simulink model "Prod_mod"  (R2016b)
settings: Solver=VariableStepAuto  StartTime=0.0  StopTime=9000  MaxStep=0.01  RelTol=1e-4  EnableMultiTasking=on
undefined symbols (not defined in the file or in its folder): DiscIntNeverNeededParam
libraries: simulink x2
settings Model: Creator=Joseph Lee  LastModifiedBy=Joseph Lee
settings DataIOCC: LimitDataPoints=on  SaveOutput=off  SaveTime=off
settings OptimizationCC: ExpressionDepthLimit=2147483647  LifeSpan=1
settings DebuggingCC: UnderspecifiedInitializationDetection=Classic  MergeDetectMultiDrivingBlocksExec=none  FcnCallInpInsideContextMsg=warning  AllowSymbolicDim=off  StateNameClashWarn=warning  SFUnexpectedBacktrackingDiag=warning  SFNoUnconditionalDefaultTransitionDiag=warning  SFExecutionAtInitializationDiag=none
settings GRTTargetCC: TargetLangStandard=C89/C90 (ANSI)  GeneratePreprocessorConditionals=Disable all  CombineOutputUpdateFcns=off  GRTInterface=on

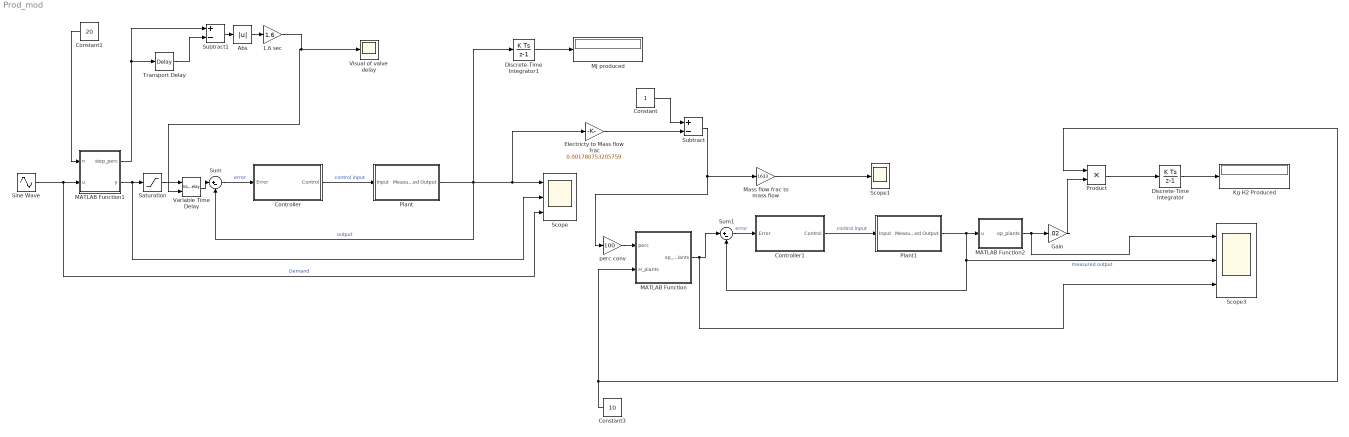
== system Prod_mod ==
  1.6 sec : Gain  Gain=1.6
  Abs : Abs  ZeroCross=off
  Constant : Constant
  Constant1 : Constant  Value=20
  Constant3 : Constant  Value=10
  Controller : Subsystem
  Controller1 : Subsystem
  Discrete-Time Integrator : DiscreteIntegrator  InitialConditionSetting=State (most efficient)  SampleTime=-1  ICPrevOutput=DiscIntNeverNeededParam  ICPrevScaledInput=DiscIntNeverNeededParam
  Discrete-Time Integrator1 : DiscreteIntegrator  InitialConditionSetting=State (most efficient)  SampleTime=-1  ICPrevOutput=DiscIntNeverNeededParam  ICPrevScaledInput=DiscIntNeverNeededParam
  "Electricty to Mass flow frac " : Gain  Gain=0.001780753205759
  Gain : Gain  Gain=.02
  Kg H2 Produced : Display
  MATLAB Function : MATLAB Function  TreatAsAtomicUnit=on
  MATLAB Function1 : MATLAB Function  TreatAsAtomicUnit=on
  MATLAB Function2 : MATLAB Function  TreatAsAtomicUnit=on
  MJ produced : Display
  "Mass flow frac to mass flow " : Gain  Gain=1633
  Plant : Subsystem
  Plant1 : Subsystem
  Product : Product
  Saturation : Saturate  UpperLimit=500  LowerLimit=0
  Scope : Scope  NumInputPorts=3
  Scope1 : Scope
  Scope3 : Scope  NumInputPorts=3
  Sine Wave : Sin  Amplitude=400  Frequency=1/300  SampleTime=0
  Subtract : Sum  Inputs=+-
  Subtract1 : Sum  Inputs=+-
  Sum : Sum  Inputs=|+-
  Sum1 : Sum  Inputs=|+-
  Transport Delay : TransportDelay
  Variable Time Delay : VariableTransportDelay  MaximumDelay=10  ZeroDelay=on
  Visual of valve delay : Scope
  perc conv : Gain  Gain=100
  wires:
  Sine Wave/1 -> Scope/3, MATLAB Function1/2(u)  "Demand"
  Plant/1(Measured Output) -> Discrete-Time Integrator1/1, "Electricty to Mass flow frac "/1, Scope/1, Sum/2  "output"
  Sum/1 -> Controller/1(Error)  "error"
  Controller/1(Control) -> Plant/1(Input)  "control input"
  "Electricty to Mass flow frac "/1 -> Subtract/2
  Constant/1 -> Subtract/1
  "Mass flow frac to mass flow "/1 -> Scope1/1
  Plant1/1(Measured Output) -> MATLAB Function2/1(u), Sum1/2, Scope3/2  "measured output"
  Sum1/1 -> Controller1/1(Error)  "error"
  Controller1/1(Control) -> Plant1/1(Input)  "control input"
  Subtract/1 -> perc conv/1, "Mass flow frac to mass flow "/1
  Constant1/1 -> MATLAB Function1/1(n)
  Variable Time Delay/1 -> Sum/1
  MATLAB Function1/2(y) -> Scope/2, Saturation/1
  Saturation/1 -> Variable Time Delay/1
  Subtract1/1 -> Abs/1
  Abs/1 -> 1.6 sec/1
  MATLAB Function1/1(step_perc) -> Transport Delay/1, Subtract1/1
  Transport Delay/1 -> Subtract1/2
  MATLAB Function/1(op_H_plants) -> Scope3/3, Sum1/1
  perc conv/1 -> MATLAB Function/1(perc)
  Constant3/1 -> MATLAB Function/2(H_plants), Product/1
  MATLAB Function2/1(op_plants) -> Scope3/1, Gain/1
  1.6 sec/1 -> Variable Time Delay/2, Visual of valve delay/1
  Gain/1 -> Product/2
  Product/1 -> Discrete-Time Integrator/1
  Discrete-Time Integrator/1 -> Kg H2 Produced/1
  Discrete-Time Integrator1/1 -> MJ produced/1

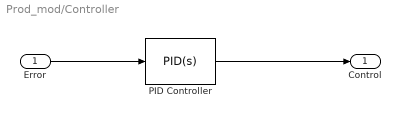
== system Prod_mod/Controller ==
  Error : Inport
  PID Controller : simulink/Continuous/PID Controller  Controller=PID  TimeDomain=Continuous-time  SampleTime=-1  IntegratorMethod=Forward Euler  FilterMethod=Forward Euler  Form=Parallel  UseFilter=on  ControllerParametersSource=internal  P=0  I=0.208323446137065  D=0  N=100  InitialConditionSource=internal  InitialConditionForIntegrator=0  InitialConditionForFilter=0  ExternalReset=none  LimitOutput=off  UpperSaturationLimit=inf  LowerSaturationLimit=-inf  LinearizeAsGain=on  AntiWindupMode=none  Kb=1  TrackingMode=off  Kt=1  PParamMin=[]  PParamMax=[]  IParamMin=[]  IParamMax=[]  DParamMin=[]  DParamMax=[]  NParamMin=[]  NParamMax=[]  KbParamMin=[]  KbParamMax=[]  KtParamMin=[]  KtParamMax=[]  POutMin=[]  POutMax=[]  IOutMin=[]  IOutMax=[]  DOutMin=[]  DOutMax=[]  NOutMin=[]  NOutMax=[]  KbOutMin=[]  KbOutMax=[]  KtOutMin=[]  KtOutMax=[]  IntegratorOutMin=[]  IntegratorOutMax=[]  FilterOutMin=[]  FilterOutMax=[]  SumOutMin=[]  SumOutMax=[]  SumI1OutMin=[]  SumI1OutMax=[]  SumI2OutMin=[]  SumI2OutMax=[]  SumI3OutMin=[]  SumI3OutMax=[]  SumDOutMin=[]  SumDOutMax=[]  SaturationOutMin=[]  SaturationOutMax=[]  IntegratorContinuousStateAttributes=''  IntegratorStateMustResolveToSignalObject=off  IntegratorRTWStateStorageClass=Auto  FilterContinuousStateAttributes=''  FilterStateMustResolveToSignalObject=off  FilterRTWStateStorageClass=Auto  DifferentiatorICPrevScaledInput=0  DifferentiatorOutMin=[]  DifferentiatorOutMax=[]
  Control : Outport
  wires:
  Error/1 -> PID Controller/1
  PID Controller/1 -> Control/1

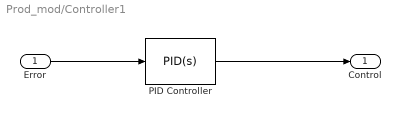
== system Prod_mod/Controller1 ==
  Error : Inport
  PID Controller : simulink/Continuous/PID Controller  Controller=PID  TimeDomain=Continuous-time  SampleTime=-1  IntegratorMethod=Forward Euler  FilterMethod=Forward Euler  Form=Parallel  UseFilter=on  ControllerParametersSource=internal  P=0  I=0.0666663426018519  D=0  N=100  InitialConditionSource=internal  InitialConditionForIntegrator=0  InitialConditionForFilter=0  ExternalReset=none  LimitOutput=off  UpperSaturationLimit=inf  LowerSaturationLimit=-inf  LinearizeAsGain=on  AntiWindupMode=none  Kb=1  TrackingMode=off  Kt=1  PParamMin=[]  PParamMax=[]  IParamMin=[]  IParamMax=[]  DParamMin=[]  DParamMax=[]  NParamMin=[]  NParamMax=[]  KbParamMin=[]  KbParamMax=[]  KtParamMin=[]  KtParamMax=[]  POutMin=[]  POutMax=[]  IOutMin=[]  IOutMax=[]  DOutMin=[]  DOutMax=[]  NOutMin=[]  NOutMax=[]  KbOutMin=[]  KbOutMax=[]  KtOutMin=[]  KtOutMax=[]  IntegratorOutMin=[]  IntegratorOutMax=[]  FilterOutMin=[]  FilterOutMax=[]  SumOutMin=[]  SumOutMax=[]  SumI1OutMin=[]  SumI1OutMax=[]  SumI2OutMin=[]  SumI2OutMax=[]  SumI3OutMin=[]  SumI3OutMax=[]  SumDOutMin=[]  SumDOutMax=[]  SaturationOutMin=[]  SaturationOutMax=[]  IntegratorContinuousStateAttributes=''  IntegratorStateMustResolveToSignalObject=off  IntegratorRTWStateStorageClass=Auto  FilterContinuousStateAttributes=''  FilterStateMustResolveToSignalObject=off  FilterRTWStateStorageClass=Auto  DifferentiatorICPrevScaledInput=0  DifferentiatorOutMin=[]  DifferentiatorOutMax=[]
  Control : Outport
  wires:
  Error/1 -> PID Controller/1
  PID Controller/1 -> Control/1

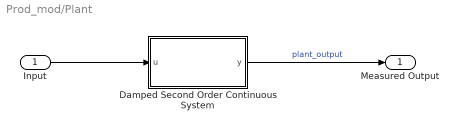
== system Prod_mod/Plant ==
  Input : Inport
  Damped Second Order Continuous System : Subsystem  mask{wn=16, zeta=0.6}
      mask prompts: wn "Undamped natural frequency (wn, rad/s)"; zeta "Damping factor (zeta)"
  Measured Output : Outport
  wires:
  Input/1 -> Damped Second Order Continuous System/1(u)
  Damped Second Order Continuous System/1(y) -> Measured Output/1  "plant_output"

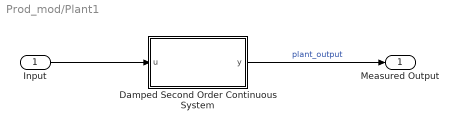
== system Prod_mod/Plant1 ==
  Input : Inport
  Damped Second Order Continuous System : Subsystem  mask{wn=16, zeta=0.6}
      mask prompts: wn "Undamped natural frequency (wn, rad/s)"; zeta "Damping factor (zeta)"
  Measured Output : Outport
  wires:
  Input/1 -> Damped Second Order Continuous System/1(u)
  Damped Second Order Continuous System/1(y) -> Measured Output/1  "plant_output"

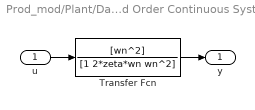
== system Prod_mod/Plant/Damped Second Order Continuous System ==
  u : Inport
  Transfer Fcn : TransferFcn  Numerator=[wn^2]  Denominator=[1 2*zeta*wn wn^2]
  y : Outport
  wires:
  Transfer Fcn/1 -> y/1
  u/1 -> Transfer Fcn/1

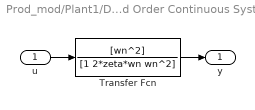
== system Prod_mod/Plant1/Damped Second Order Continuous System ==
  u : Inport
  Transfer Fcn : TransferFcn  Numerator=[wn^2]  Denominator=[1 2*zeta*wn wn^2]
  y : Outport
  wires:
  Transfer Fcn/1 -> y/1
  u/1 -> Transfer Fcn/1

== matlab function Prod_mod/MATLAB Function1 ==
  data: n input; step_perc output; u input; y output
function [step_perc,y] = fcn(n,u)
N=500/n;
step_perc=ceil(u/N)/N;
y = N*ceil(u/N);

== matlab function Prod_mod/MATLAB Function ==
  data: perc input; op_H_plants output; H_plants input
function op_H_plants = fcn(perc,H_plants)
interval=100/H_plants;
op_H_plants=floor(perc/interval);

== matlab function Prod_mod/MATLAB Function2 ==
  data: u input; op_plants output
function op_plants = fcn(u)
op_plants=floor(u+.001);
